simulink model "model1"  (R2022a)
settings: Solver=VariableStepAuto  StartTime=0.0  StopTime=10  RelTol=1e-3
PreLoadFcn:
  | m = 3.600;     % kg
  | k = 400;    % N/m
  | b = 10;      % Ns/m
  | x0=1; %m
settings Model: Creator=whatastarrynight  LastModifiedBy=Tsing

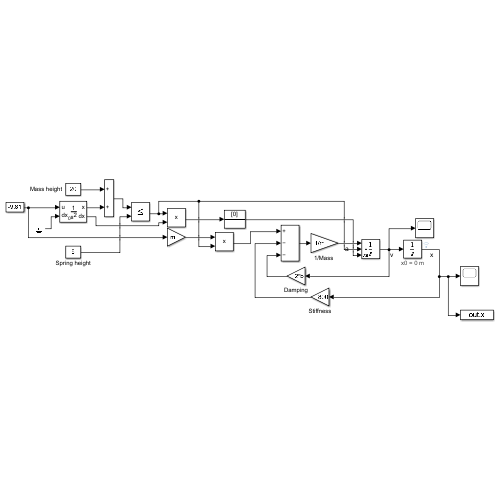
[thumbnail: Simulink's stored preview of the top-level diagram]
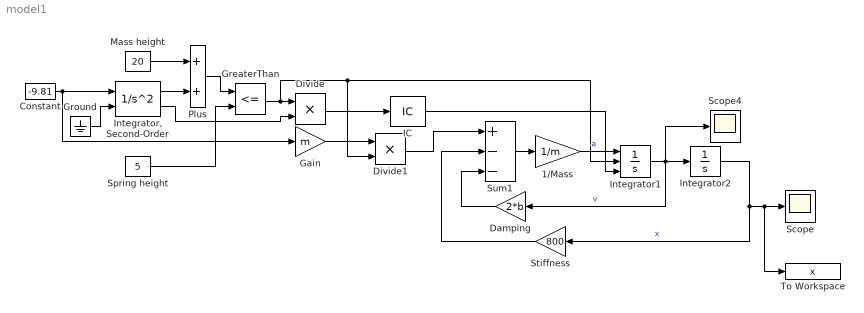
== system model1 ==
  "1/Mass " : Gain  Gain=1/m  SaturateOnIntegerOverflow=on  OutDataTypeStr=Inherit: Same as input  ParamDataTypeStr=Inherit: Same as input
  Constant : Constant  Value=-9.81
  Damping : Gain  Gain=2*b  SaturateOnIntegerOverflow=on  OutDataTypeStr=Inherit: Same as input  ParamDataTypeStr=Inherit: Same as input
  Divide : Product  Inputs=**
  Divide1 : Product  Inputs=**
  Gain : Gain  Gain=m
  GreaterThan : RelationalOperator  Operator=<=  OutDataTypeStr=boolean  RndMeth=Simplest  InputSameDT=off
  Ground : Ground
  IC : InitialCondition  Value=0
  "Integrator, Second-Order" : SecondOrderIntegrator  ICSourceDXDT=external
  Integrator1 : Integrator  ExternalReset=rising  InitialConditionSource=external
  Integrator2 : Integrator
      settings: AttributesFormatString=x0 = %<InitialCondition> m
  Mass height : Constant  Value=20
  Plus : Sum
  Scope : Scope
  Scope4 : Scope
  Spring height : Constant  Value=5
  Stiffness : Gain  Gain=800  SaturateOnIntegerOverflow=on  OutDataTypeStr=Inherit: Same as input  ParamDataTypeStr=Inherit: Same as input
  Sum1 : Sum  Inputs=+--  InputSameDT=on  SaturateOnIntegerOverflow=on  OutDataTypeStr=Inherit: Same as first input
  To Workspace : ToWorkspace  VariableName=x  SaveFormat=Timeseries  SampleTime=-1
  wires:
  Stiffness/1 -> Sum1/2
  Sum1/1 -> "1/Mass "/1
  Integrator2/1 -> To Workspace/1, Scope/1, Stiffness/1  "x"
  "1/Mass "/1 -> Integrator1/1  "a"
  Damping/1 -> Sum1/3
  Integrator1/1 -> Scope4/1, Integrator2/1, Damping/1  "v"
  Mass height/1 -> Plus/1
  Constant/1 -> "Integrator, Second-Order"/1, Gain/1
  "Integrator, Second-Order"/1 -> Plus/2
  Plus/1 -> GreaterThan/1
  Spring height/1 -> GreaterThan/2
  "Integrator, Second-Order"/2 -> Divide/2
  Divide/1 -> IC/1
  Ground/1 -> "Integrator, Second-Order"/2
  GreaterThan/1 -> Divide1/2, Integrator1/2, Divide/1
  IC/1 -> Integrator1/3
  Divide1/1 -> Sum1/1
  Gain/1 -> Divide1/1
